simulink model "Model_Linearisierung_final"  (R2023b)
settings: Solver=FixedStepAuto  StartTime=0.0  StopTime=Inf  FixedStep=1e-4  RelTol=1e-3
PostLoadFcn:
  | if any(exist('dsrtsu_mdlpostloadfcn', 'file') ~= 0), dsrtsu_mdlpostloadfcn('Execute', bdroot); end
InitFcn:
  | , if any(exist('rtifpga_mdlclblib', 'file') ~= 0), rtifpga_mdlclblib('Init', bdroot); end,
  | , if any(exist('dsmpb_private', 'file') ~= 0), dsmpb_private('dsmpb_mdlclblib', 'Init', bdroot); end,
  | load('LUT_BRUSA_jax_grad.mat')
  | load('daten_nichtlinear_interpoliert.mat')
  | load('Maschinendaten.mat')
values from neighbouring files (symbols this model uses):
  delta_id = id_fine(2)-id_fine(1)    [Messdaten_Interpoliert.m]    (also in daten_nichtlinear_interpoliert.mat = 2.52525252525)
  delta_iq = iq_fine(2)-iq_fine(1)    [Messdaten_Interpoliert.m]    (also in daten_nichtlinear_interpoliert.mat = 5.05050505051)
  I_max = 170    [Maschinendaten.mat]    (also in Maschinendaten_Vorgabe.m; test_ModelParameters.m = evalin('base', 'I_max'); test_StrategySelection.m = tc.readConstant(tc.BLK_Imax))
  ID = [-250 -250 -250 -250 -250 -250 -250 -250 -250 -250 -250 -250 ... (10000 elements, 100x100)]    [daten_nichtlinear_interpoliert.mat]
  id_fine = linspace(min(id_vec), max(id_vec), 100)    [Messdaten_Interpoliert.m]    (also in daten_nichtlinear_interpoliert.mat = [-250 -247.474747475 -244.949494949 -242.424242424 -239.8989)
  IQ = [-250 -244.949494949 -239.898989899 -234.848484848 -229.797979798 -224.747474747 -219.696969697 -214.646464646 -209.595959596 -204.545454545 -199.494949495 -194.444444444 ... (10000 elements, 100x100)]    [daten_nichtlinear_interpoliert.mat]
  iq_fine = linspace(min(iq_vec), max(iq_vec), 100)    [Messdaten_Interpoliert.m]    (also in daten_nichtlinear_interpoliert.mat = [-250 -244.949494949 -239.898989899 -234.848484848 -229.7979)
  Ldd = Ldd_fine    [Messdaten_Interpoliert.m]    (also in daten_nichtlinear_interpoliert.mat = [0.000225276031415 0.000225750625371 0.000226241749969 0.000)
  Ldq = Ldq_fine    [Messdaten_Interpoliert.m]    (also in daten_nichtlinear_interpoliert.mat = [1.31113456519e-05 1.34236782585e-05 1.31001168558e-05 1.236)
  Lqd = Lqd_fine    [Messdaten_Interpoliert.m]    (also in daten_nichtlinear_interpoliert.mat = [7.22855329514e-05 7.00325573553e-05 6.7613098921e-05 6.5016)
  Lqq = Lqq_fine    [Messdaten_Interpoliert.m]    (also in daten_nichtlinear_interpoliert.mat = [0.000286039721686 0.000286453471045 0.000286025480511 0.000)
  n_max = 11000    [Maschinendaten.mat]    (also in Maschinendaten_Vorgabe.m; test_ModelParameters.m = evalin('base', 'n_max'); test_StrategySelection.m = tc.readConstant(tc.BLK_nmax))
  p = 3    [Maschinendaten.mat]    (also in Maschinendaten_Vorgabe.m; Messdaten_Interpoliert.m; test_ModelParameters.m = evalin('base', 'p'))
  Psid = Psid_fine    [Messdaten_Interpoliert.m]    (also in daten_nichtlinear_interpoliert.mat = [0.00602681114795 0.00609490588107 0.00615917040906 0.006219)
  Psiq = Psiq_fine    [Messdaten_Interpoliert.m]    (also in daten_nichtlinear_interpoliert.mat = [-0.166252688687 -0.164805403122 -0.163363500753 -0.16192610)
  Rs = 0.018    [Maschinendaten.mat]    (also in Maschinendaten_Vorgabe.m; test_ModelParameters.m = evalin('base', 'Rs'))
  U_dc = 560    [Maschinendaten.mat]    (also in Maschinendaten_Vorgabe.m; test_ModelParameters.m = evalin('base', 'U_dc'))
  U_max = 323.316150746    [Maschinendaten.mat]    (also in Maschinendaten_Vorgabe.m = U_dc / sqrt(3); test_ModelParameters.m = evalin('base', 'U_max'))
(part 2 of 3)

== matlab function Model_Linearisierung_final/Subsystem Arbeitspunktsteuerung/Arbeitspunktsteuerung/Glac - Schnittpunktsuche ==
  data: q_current input double size=[1 6]; q_voltage input double size=[1 6]; q_torque input size=[1 6]; q_MTPC input double size=[1 6]; q_MTPV input double size=[1 6]; Imax input size=1; i_ac output size=[4 2]; i_vv output size=[4 2]; i_av output size=[4 2]; i_cv output size=[4 2]; i_at output size=[4 2]; i_tv output size=[4 2]
function [i_ac, i_vv, i_av, i_cv, i_at, i_tv] = ...
    Glac_Block(q_current, q_voltage, q_torque, q_MTPC, q_MTPV, Imax)

%#codegen
coder.extrinsic('disp');
% ================================================================
% GLAC – Schnittpunktbestimmung zweier Quadriken
%
% Eingänge:
%   q_current : Stromkreis
%   q_voltage : Spannungsgrenze
%   q_torque  : Drehmomentkennlinie
%   q_MTPC    : MTPC
%   q_MTPV    : MTPV
%   Imax      : maximaler Strom
%
% Jede Quadrik:
%   q = [a b c d e f]
%
% F(id,iq) =
%   a*id^2 + b*id*iq + c*iq^2 + d*id + e*iq + f
%
% Ausgänge:
%   jeweils 4x2
%
%   [id1 iq1
%    id2 iq2
%    id3 iq3
%    id4 iq4]
%
% Nicht vorhandene Schnittpunkte = NaN
% ================================================================


%% 1. Schnittpunkte bestimmen

% MTPC ∩ Stromkreis
i_ac = intersectGlac(q_MTPC, q_current, Imax);

% MTPV ∩ Spannung
i_vv = intersectGlac(q_MTPV, q_voltage, Imax);

% MTPC ∩ Spannung
i_av = intersectGlac(q_MTPC, q_voltage, Imax);

% Stromkreis ∩ Spannung
i_cv = intersectGlac(q_current, q_voltage, Imax);

% MTPC ∩ Drehmoment
i_at = intersectGlac(q_MTPC, q_torque, Imax);

% Drehmoment ∩ Spannung
i_tv = intersectGlac(q_torque, q_voltage, Imax);

disp('--- Schnittpunkte: i_ac, i_vv, i_av, i_cv, i_at, i_tv ---');
disp('i_ac:');
disp(i_ac);
disp('i_vv:');
disp(i_vv);
disp('i_av:');
disp(i_av);
disp('i_cv:');
disp(i_cv);
disp('i_at:');
disp(i_at);
disp('i_tv:');
disp(i_tv);
end

%%%%%%%%%%%%%%%%%%%%%%%%%%%%%%%%%%%%%%%%%%%%%%%%%%%%%%%%%%%%%%%%%%%%%%%%%%%
%% GLAC-SCHNITTPUNKTSUCHE ==> Überprüft !
% Analytische Schnittpunktbestimmung zweier Quadriken nach Glac
%
% Eingabe:
%   qA, qB : Quadrikkoeffizienten [a b c d e f]
%            F(id, iq) = a*id^2 + b*id*iq + c*iq^2 + d*id + e*iq + f = 0
%   Imax   : Maximaler Strom zur Normierung [A]
%
% Ausgabe:
%   pts    : 4x2 Matrix mit [id, iq]-Schnittpunkten, sortiert nach
%            dem Glac-Gütefaktor s = idN^2 + 0.1*iqN^2.
%            Nicht existierende Schnittpunkte sind mit NaN befüllt.

function pts = intersectGlac(qA, qB, Imax)

    % ---Ausgabe immer 4x2 ---------------------------------------------------
    pts = NaN(4, 2);
    ZERO_TOL = 1e-12; % Glac Toleranz für Null-Konstante 9.0e-4 -> ggf 1e-10

    %% 1. Normierung der Quadriken auf Imax
    A = zeros(1, 6);
    B = zeros(1, 6);
    A(1) = qA(1); 
    A(2) = qA(2); 
    A(3) = qA(3); 
    A(4) = qA(4)/Imax; 
    A(5) = qA(5)/Imax; 
    A(6) = qA(6)/(Imax*Imax);
    B(1) = qB(1); 
    B(2) = qB(2); 
    B(3) = qB(3); 
    B(4) = qB(4)/Imax; 
    B(5) = qB(5)/Imax; 
    B(6) = qB(6)/(Imax*Imax);

    %% 2. Transformation in Glac-Matrixdarstellung
    % F = x11*x1^2 + 2*x12*x1*x2 + x22*x2^2 + 2*x1*x1 + 2*x2*x2 + x0
    M_A_x11 = A(1); 
    M_A_x12 = A(2)/2; 
    M_A_x22 = A(3); 
    M_A_x1  = A(4)/2; 
    M_A_x2  = A(5)/2; 
    M_A_x0  = A(6);

    M_B_x11 = B(1); 
    M_B_x12 = B(2)/2; 
    M_B_x22 = B(3); 
    M_B_x1  = B(4)/2; 
    M_B_x2  = B(5)/2; 
    M_B_x0  = B(6);


    %% 3. Fallunterscheidung zur Bildung der Matrizen D und M
    translate = false;

    if (abs(M_A_x0) > ZERO_TOL) && (abs(M_B_x0) > ZERO_TOL)
        % Fall 1: Beide Konstantenterme != 0
        a0inv = 1 / M_A_x0;
        b0inv = 1 / M_B_x0;

        D_x11 = M_A_x11*a0inv - M_B_x11*b0inv;
        D_x12 = M_A_x12*a0inv - M_B_x12*b0inv;
        D_x22 = M_A_x22*a0inv - M_B_x22*b0inv;
        D_x1  = M_A_x1*a0inv  - M_B_x1*b0inv;
        D_x2  = M_A_x2*a0inv  - M_B_x2*b0inv;

        if abs(a0inv) > abs(b0inv)
            M_x11 = M_B_x11; M_x12 = M_B_x12; M_x22 = M_B_x22;
            M_x1  = M_B_x1;  M_x2  = M_B_x2;  M_x0  = M_B_x0;
        else
            M_x11 = M_A_x11; M_x12 = M_A_x12; M_x22 = M_A_x22;
            M_x1  = M_A_x1;  M_x2  = M_A_x2;  M_x0  = M_A_x0;
        end

    elseif (abs(M_A_x0) <= ZERO_TOL) && (abs(M_B_x0) > ZERO_TOL)
        % Fall 2: A.x0 == 0, B.x0 != 0
        D_x11 = M_A_x11; D_x12 = M_A_x12; D_x22 = M_A_x22;
        D_x1  = M_A_x1;  D_x2  = M_A_x2;
        M_x11 = M_B_x11; M_x12 = M_B_x12; M_x22 = M_B_x22;
        M_x1  = M_B_x1;  M_x2  = M_B_x2;  M_x0  = M_B_x0;

    elseif (abs(M_A_x0) > ZERO_TOL) && (abs(M_B_x0) <= ZERO_TOL)
        % Fall 3: A.x0 != 0, B.x0 == 0
        D_x11 = M_B_x11; D_x12 = M_B_x12; D_x22 = M_B_x22;
        D_x1  = M_B_x1;  D_x2  = M_B_x2;
        M_x11 = M_A_x11; M_x12 = M_A_x12; M_x22 = M_A_x22;
        M_x1  = M_A_x1;  M_x2  = M_A_x2;  M_x0  = M_A_x0;

    else
        % Fall 4: Beide x0 == 0 -> Translation
        xs1 = 0.5;
        xs2 = 0.3;

        alfa_s = 2*M_A_x1*xs1 + 2*M_A_x2*xs2 + ...
                 xs1*(M_A_x11*xs1 + M_A_x12*xs2) + ...
                 xs2*(M_A_x12*xs1 + M_A_x22*xs2);

        beta_s = 2*M_B_x1*xs1 + 2*M_B_x2*xs2 + ...
                 xs1*(M_B_x11*xs1 + M_B_x12*xs2) + ...
                 xs2*(M_B_x12*xs1 + M_B_x22*xs2);

        if abs(alfa_s) < 1e-12 || abs(beta_s) < 1e-12
            return;
        end

        alfa_s_inv = 1 / alfa_s;
        beta_s_inv = 1 / beta_s;

        D_x11 = M_A_x11*alfa_s_inv - M_B_x11*beta_s_inv;
        D_x12 = M_A_x12*alfa_s_inv - M_B_x12*beta_s_inv;
        D_x22 = M_A_x22*alfa_s_inv - M_B_x22*beta_s_inv;

        D_x1 = (M_A_x1 + M_A_x11*xs1 + M_A_x12*xs2)*alfa_s_inv - ...
               (M_B_x1 + M_B_x11*xs1 + M_B_x12*xs2)*beta_s_inv;

        D_x2 = (M_A_x2 + M_A_x12*xs1 + M_A_x22*xs2)*alfa_s_inv - ...
               (M_B_x2 + M_B_x12*xs1 + M_B_x22*xs2)*beta_s_inv;

        M_x11 = M_B_x11; M_x12 = M_B_x12; M_x22 = M_B_x22;
        M_x1  = M_B_x1 + M_B_x11*xs1 + M_B_x12*xs2;
        M_x2  = M_B_x2 + M_B_x12*xs1 + M_B_x22*xs2;
        M_x0  = beta_s;

        translate = true;
    end

    if abs(M_x0) < 1e-14
        return;
    end


 %% 4. Aufstellen des Quartik-Polynoms in xi
    invM0 = 1 / M_x0;
    xi4 = 1.0;
    xi3 = invM0 * (4*D_x2*M_x1 - 4*D_x1*M_x2);
    xi2 = invM0 * (4*D_x2^2*M_x11 + 4*D_x1^2*M_x22 - 2*D_x12^2*M_x0 ...
                 - 8*D_x1*D_x2*M_x12 + 4*D_x1*D_x12*M_x2 - 4*D_x2*D_x11*M_x2 ...
                 + 4*D_x2*D_x12*M_x1 - 4*D_x1*D_x22*M_x1 + 2*D_x11*D_x22*M_x0);
    xi1 = invM0 * (4*D_x1*D_x12^2*M_x2 - 4*D_x2*D_x12^2*M_x1 ...
                 - 8*D_x2^2*D_x11*M_x12 + 8*D_x2^2*D_x12*M_x11 ...
                 - 8*D_x1^2*D_x12*M_x22 + 8*D_x1^2*D_x22*M_x12 ...
                 + 8*D_x1*D_x2*D_x11*M_x22 - 8*D_x1*D_x2*D_x22*M_x11 ...
                 - 4*D_x1*D_x11*D_x22*M_x2 + 4*D_x2*D_x11*D_x22*M_x1);
    xi0 = invM0 * (D_x12^4*M_x0 + 4*D_x2^2*D_x12^2*M_x11 + 4*D_x1^2*D_x22^2*M_x11 ...
                 + 4*D_x1^2*D_x12^2*M_x22 + 4*D_x2^2*D_x11^2*M_x22 + D_x11^2*D_x22^2*M_x0 ...
                 - 4*D_x1*D_x12^3*M_x2 - 4*D_x2*D_x12^3*M_x1 + 8*D_x1*D_x2*D_x12^2*M_x12 ...
                 + 4*D_x2*D_x11*D_x12^2*M_x2 - 4*D_x1*D_x11*D_x22^2*M_x1 ...
                 + 4*D_x1*D_x12^2*D_x22*M_x1 - 4*D_x2*D_x11^2*D_x22*M_x2 ...
                 - 8*D_x2^2*D_x11*D_x12*M_x12 - 8*D_x1^2*D_x12*D_x22*M_x12 ...
                 - 2*D_x11*D_x12^2*D_x22*M_x0 - 8*D_x1*D_x2*D_x11*D_x12*M_x22 ...
                 + 8*D_x1*D_x2*D_x11*D_x22*M_x12 - 8*D_x1*D_x2*D_x12*D_x22*M_x11 ...
                 + 4*D_x1*D_x11*D_x12*D_x22*M_x2 + 4*D_x2*D_x11*D_x12*D_x22*M_x1);

 

    %% 5. Quartik lösen
    xiRoots = roots([xi4, xi3, xi2, xi1, xi0]);
    
    disp('xiRoots:');
    disp(xiRoots);

    %% 6. Rekonstruktion der Schnittpunkte (id, iq)
    validCount = 0;
    tempPts = NaN(4, 2);
    tempSort = NaN(4, 1);

    for k = 1:numel(xiRoots)
        xi = xiRoots(k);

        % Nur reelle Nullstellen verarbeiten
        if abs(imag(xi)) < 1e-6
            xi_r = real(xi);
            denXi = xi_r^2 + D_x11*D_x22 - D_x12^2;

            if abs(denXi) > 1e-12
                adjXi = 1 / denXi;

                if translate
                    xs1 = 0.5; xs2 = 0.3;
                    idN = -2*adjXi*(D_x22*D_x1 + (-D_x12 - xi_r)*D_x2) + xs1;
                    iqN = -2*adjXi*((xi_r - D_x12)*D_x1 + D_x11*D_x2) + xs2;
                else
                    idN = -2*adjXi*(D_x22*D_x1 + (-D_x12 - xi_r)*D_x2);
                    iqN = -2*adjXi*((xi_r - D_x12)*D_x1 + D_x11*D_x2);
                end

                if abs(imag(idN)) < 1e-6 && abs(imag(iqN)) < 1e-6
                    idN = real(idN);
                    iqN = real(iqN);

                    id = idN * Imax;
                    iq = iqN * Imax;

                    % Residuen-Prüfung gegen ursprüngliche Quadriken
                    resA = qA(1)*id^2 + qA(2)*id*iq + qA(3)*iq^2 + qA(4)*id + qA(5)*iq + qA(6);
                    resB = qB(1)*id^2 + qB(2)*id*iq + qB(3)*iq^2 + qB(4)*id + qB(5)*iq + qB(6);
                    
                    scaleA = abs(qA(1)*id^2) + abs(qA(2)*id*iq) + abs(qA(3)*iq^2) + abs(qA(4)*id) + abs(qA(5)*iq) + abs(qA(6)) + 1;
                    scaleB = abs(qB(1)*id^2) + abs(qB(2)*id*iq) + abs(qB(3)*iq^2) + abs(qB(4)*id) + abs(qB(5)*iq) + abs(qB(6)) + 1;

                    disp('xi =');
                    disp(xi_r);
                    disp('idN =');
                    disp(idN);
                    disp(' iqN =');
                    disp(iqN);
                    disp('resA = ');
                    disp(abs(resA)/scaleA);
                    disp('resB = ');
                    disp(abs(resB)/scaleB);

                    if (abs(resA)/scaleA < 1e-2) && (abs(resB)/scaleB < 1e-2)
                        validCount = validCount + 1;
                        tempPts(validCount, :) = [id, iq];
                        tempSort(validCount) = idN^2 + 0.1*iqN^2; % Glac Sortierkriterium
                    end
                end
            end
        end
    end

    %% 7. Aufsteigend nach Glac-Gütekriterium sortieren
    if validCount > 0
        [~, idx] = sort(tempSort(1:validCount), 'ascend');
        for i = 1:validCount
            pts(i, :) = tempPts(idx(i), :);
        end
    end
end

== matlab function Model_Linearisierung_final/Subsystem Arbeitspunktsteuerung/Vorläufiger Arbeitspunkt aus alter Steuerug/Kennfelder/ Vorberechnung gemeinsamer Größen ==
  data: ID input; IQ input; Ld input; Lq input; Lm input; PSID input; PSIQ input; Rs input; omega input; p input; I_max input; U_max input; Ldq output; Ldq_p output; Ld_q output; Lq_d output; Ld2 output; Lq2 output; Lm2 output; psid1 output; psiq1 output; omega2 output; Rs2 output; stromgrenze output; spannungsgrenze output; I_max2 output; U_max2 output; psi2 output; T_ref output; T_feld output; T_soll input
%% 4) Vorberechnung gemeinsamer Größen
% Dieser Block dient der Laufzeitoptimierung.
% Alle häufig benötigten Terme werden einmal zentral berechnet und später
% wiederverwendet. So werden Mehrfachrechnungen vermieden.

function [Ldq, Ldq_p, Ld_q, Lq_d, Ld2, Lq2, Lm2, psid1, psiq1, omega2, Rs2, stromgrenze, spannungsgrenze, I_max2, U_max2, psi2, T_ref, T_feld] = fcn(ID, IQ, Ld, Lq, Lm, PSID, PSIQ, Rs, omega, p, I_max, U_max, T_soll)

% Strom und Spannungsgrenzen
ID2   = ID.^2;
IQ2   = IQ.^2;
IDIQ  = ID.*IQ;

% Maschinenparameter
Ldq = Ld - Lq;      % Differenz Ld - Lq
Ldq_p = Ld + Lq;    % Summe Ld + Lq
Ld_q = Ld.*Lq;      % Matrixmultiplikation Ld.* Lq
Lq_d = Lq.*Ld;      % Matrixmultiplikation Lq.* Ld
Ld2 = Ld.^2;        % Quadrat Ld
Lq2 = Lq.^2;        % Quadrat Lq
Lm2 = Lm.^2;        % Quadrat Lm
psid1 = 1.5*p*PSID; % Vorfaktor PSID
psiq1 = 1.5*p*PSIQ; % Vorfaktor PSIQ
omega2 = omega^2;   % Quadrat Omega
Rs2 = Rs^2;         % Quadrat Rs

% Spannungsanteile in d- und q-Richtung
ud = Rs .* ID - omega .* PSIQ;
uq = Rs .* IQ + omega .* PSID;

% Quadrat von Strom- und Spannungsbetrag
I2 = ID2 + IQ2;
U2 = ud.^2 + uq.^2;

I_max2 = I_max^2;
U_max2 = U_max^2;

% Grenzfunktionen:
stromkreis = I2 - I_max2; % Stromkreis (Betragsgrenze)
spannung   = U2 - U_max2; % Spannungsellipse
stromgrenze = stromkreis;
spannungsgrenze = spannung;

% Flussbetrag
psi2 = PSID.^2 + PSIQ.^2;

% Drehmoment
T_feld = 3/2*p*(PSID.*IQ - PSIQ.*ID);

% Referenz-Drehmomenthyperbel
T_ref = T_feld - T_soll;

== matlab function Model_Linearisierung_final/Subsystem Arbeitspunktsteuerung/Vorläufiger Arbeitspunkt aus alter Steuerug/Kennfelder/MTPC-Kennlinie ==
  data: psid1 input; psiq1 input; Lm input; f_MTPC output; Ldq input; p input; ID input; IQ input
%% MTPC Kennlinie 
% konstant, da nur abhängig von Induktivitäten und Flüssen  
function f_MTPC = fcn(psid1, psiq1, Lm, Ldq, p, ID, IQ)

%Psi_pm = 0.068; 
M11 = (Ldq)./2;
M12 = Lm;
M22 = -(Ldq)./2;
mc1 = psid1./4;
mc2 = psiq1./4;

f_MTPC = 1.5*p*(M11.*ID.^2 + 2*M12.*ID.*IQ + M22.*IQ.^2)...
         + 2*(mc1.*ID + mc2.*IQ);

== matlab function Model_Linearisierung_final/Subsystem Arbeitspunktsteuerung/Vorläufiger Arbeitspunkt aus alter Steuerug/Kennfelder/MTPF-Kennlinie ==
  data: Lm input; f_MTPF output; Ld input; Lq input; Ldq input; Ldq_p input; Ld2 input; Lq2 input; Ld_q input; Lq_d input; Lm2 input; PSID input; PSIQ input; p input; ID input; IQ input
%% MTPF Kennlinie 
% konstant, da nur abhängig von Induktivitäten und Flüssen
function f_MTPF = fcn(Lm, Ld, Lq, Ldq, Ldq_p, Ld2, Lq2, Ld_q, Lq_d, Lm2, PSID, PSIQ, p, ID, IQ)

Mf11 = (Ldq)./2 .*(Ld2 + Lm2) + Lm2 .*(Ldq_p);
Mf12 = Lm./2.*(Ld2 + Lq2 + 2*Lm2);
Mf22 = -(Ldq)./2 .*(Lq2 + Lm2) + Lm2 .*(Ldq_p);

mf1 = 1.5*p*((2*Ld2 - Lq_d + 3*Lm2).*PSID./4 ...
      + Lm.* (Ldq_p).*PSIQ./2);
mf2 = 1.5*p*(Lm.* (Ldq_p).*PSID./2 ...
      + (2*Lq2 - Ld_q + 3*Lm2).*PSIQ./4);

my_f = 0.75*p*(Ld.*(PSID).^2 + 2*Lm.*PSID.*PSIQ + Lq.*(PSIQ).^2);

f_MTPF = 1.5*p*(Mf11.*ID.^2 + 2*Mf12.*ID.*IQ + Mf22.*IQ.^2)...
         + 2*(mf1.*ID + mf2.*IQ) + my_f;

== matlab function Model_Linearisierung_final/Subsystem Arbeitspunktsteuerung/Vorläufiger Arbeitspunkt aus alter Steuerug/Kennfelder/MTPV-Kennlinie ==
  data: Lm input; f_MTPV output; Ld input; Lq input; Lm2 input; Ld2 input; Lq2 input; Ldq input; Ldq_p input; Lq_d input; PSID input; PSIQ input; p input; omega2 input; ID input; IQ input; Rs2 input
%% MTPV Kennlinie 
% Ändert sich mit Drehzahl omega
function f_MTPV = fcn(Lm, Ld, Lq, Lm2, Ld2, Lq2, Ldq, Ldq_p, Lq_d, PSID, PSIQ, p, omega2, ID, IQ, Rs2)

Mv11 = omega2*Lm2.*(Ldq_p)...
       + (Ldq)./2 .*(Rs2 + omega2*(Ld2 + Lm2));
Mv12 = Lm./2.*(2*Rs2+omega2*(Ld2 + Lq2 + 2*Lm2));
Mv22 = omega2*Lm2.*(Ldq_p)...
       - (Ldq)./2 .*(Rs2 + omega2*(Lq2 + Lm2));
mv1 = 1.5*p*((Rs2 + omega2* (2*Ld2 - Lq_d + 3*Lm2)).*PSID./4 ... 
      + omega2*Lm.* (Ldq_p).*PSIQ./2);
mv2 = 1.5*p*(omega2*Lm.* (Ldq_p).*PSID./2 ...
      + (Rs2 + omega2*(2*Ld2 - Lq_d + 3*Lm2)).*PSIQ./4);
my_v = 0.75*p*omega2*(Ld.*(PSID).^2 + 2*Lm.*PSID.*PSIQ + Lq.*(PSIQ).^2);

f_MTPV = 1.5*p*(Mv11.*ID.^2 + 2*Mv12.*ID.*IQ + Mv22.*IQ.^2)...
         + 2*(mv1.*ID + mv2.*IQ) + my_v;

== matlab function Model_Linearisierung_final/Subsystem Arbeitspunktsteuerung/Vorläufiger Arbeitspunkt aus alter Steuerug/Strategieauswahl und Arbeitspunkt id*, iq* ==
  data: n_mech input; n_max input; T_soll input; T_feld input; T_ref input; signT input; id_fine input; iq_fine input; I_max2 input; U_max2 input; stromkreis input; spannung input; psi2 input; f_MTPC input; f_MTPV input; f_MTPF input; id_ref output; iq_ref output; out_iat output; out_itv output; out_iac output; out_icv output; feasCode output; boundaryCode output
%% Strategieauswahl gemäß Flowchart und Bestimmung Arbeitspunkt id*, iq*
% Interpolation, Charak. Punkte, Flowchart-Logik, Nachverfeinerung

function [id_ref, iq_ref, out_iat, out_itv, out_iac, out_icv, feasCode, boundaryCode] = fcn( ...
     n_mech, n_max, T_soll, T_feld, T_ref, signT,...
     id_fine, iq_fine, I_max2, U_max2, ...
     stromkreis,spannung, psi2, f_MTPC, f_MTPV, f_MTPF)

% Strategiecodes, da keine Textausgabe möglich:
% Fälle:
%   out_iat = 1  -> MTPC ∩ T_soll, Sollmoment erreichbar
%   out_itv = 1  -> U_max ∩ T_soll, Sollmoment erreichbar
%   out_iac = 1  -> MTPC ∩ I_max, Sollmoment nicht erreichbar
%   out_icv = 1  -> I_max ∩ U_max, Sollmoment nicht erreichbar
%
% feasCode:
% 0 = none
% 1 = i_vv
% 2 = i_ac
% 3 = i_cv
%
% boundaryCode:
% 0 = none
% 1 = voltage boundary
% 2 = current boundary

%% Konstanten fuer Root-/Mode-Codes
ROOT_AC = 1;
ROOT_VV = 2;
ROOT_AV = 3;
ROOT_CV = 4;
ROOT_AT = 5;
ROOT_TV = 6;

MODE_INTERIOR = 1;
MODE_BOUNDARY = 2;
MODE_VOLTAGE  = 3;

BND_NONE    = 0;
BND_VOLTAGE = 1;
BND_CURRENT = 2;

%% Initialisierung
id_ref = 0.0;
iq_ref = 0.0;
feasCode = int32(0);
boundaryCode = int32(0);

i_ref  = [NaN NaN];
i_feas = [NaN NaN];

out_iat = 0.0;
out_itv = 0.0;
out_iac = 0.0;
out_icv = 0.0;

%% Schutz
if n_mech > n_max
    id_ref = 0.0;
    iq_ref = 0.0;
    feasCode = int32(0);
    boundaryCode = int32(0);
    return;
end

%% 4) Kontext
ctx.xvec   = id_fine;
ctx.yvec   = iq_fine;
ctx.Ti     = T_feld;
ctx.Teql   = T_ref;
ctx.Ieql   = stromkreis;
ctx.Ueql   = spannung;
ctx.Psi2i  = psi2;
ctx.MTPCi  = f_MTPC;
ctx.MTPVi  = f_MTPV;
ctx.MTPFi  = f_MTPF;
ctx.Tref   = T_soll;
ctx.signT  = signT;
ctx.tolEq  = 1e-6 * max([1, I_max2, U_max2, abs(T_soll)]);
ctx.tolT   = max(0.25, 1e-3*max(1, abs(T_soll)));

%% 5) Charakteristische Punkte im Flowchart
pts_iac = findCurveIntersections(id_fine, iq_fine, f_MTPC,    0.0, stromkreis, 0.0, ctx);
pts_ivv = findCurveIntersections(id_fine, iq_fine, f_MTPV,    0.0, spannung,   0.0, ctx);
pts_iav = findCurveIntersections(id_fine, iq_fine, f_MTPC,    0.0, spannung,   0.0, ctx);
pts_icv = findCurveIntersections(id_fine, iq_fine, stromkreis,0.0, spannung,   0.0, ctx);
pts_iat = findCurveIntersections(id_fine, iq_fine, f_MTPC,    0.0, T_ref,  0.0, ctx);
pts_itv = findCurveIntersections(id_fine, iq_fine, T_ref, 0.0, spannung,   0.0, ctx);

i_ac = chooseCorrectRoot(pts_iac, ROOT_AC, ctx);
i_vv = chooseCorrectRoot(pts_ivv, ROOT_VV, ctx);
i_av = chooseCorrectRoot(pts_iav, ROOT_AV, ctx);
i_cv = chooseCorrectRoot(pts_icv, ROOT_CV, ctx);
i_at = chooseCorrectRoot(pts_iat, ROOT_AT, ctx);
i_tv = chooseCorrectRoot(pts_itv, ROOT_TV, ctx);

%% 6) Flowchart-Logik
% ------------------------------------------------------------
% Fall 1: MTPC ∩ T_soll -> i_at
% Nur wenn Sollmoment auf dem MTPC-Zweig noch erreichbar ist
% ------------------------------------------------------------

if isFinitePoint(i_at)
    I_at = evalGI(ctx.Ieql, i_at, ctx);
    U_at = evalGI(ctx.Ueql, i_at, ctx);

    if (I_at <= 1e-5) && (U_at <= 1e-5)
        i_ref = finalFeasiblePolish(i_at, MODE_INTERIOR, ctx);
        out_iat = 1;    % Sollmoment T* auf MTPC
    end
end

% --- falls MTPC ∩ T_soll nicht direkt zulässig ---
if ~isFinitePoint(i_ref)
    % i_feas bestimmen:
    % Vergleich psi_cv und psi_ac:
    %    - psi_cv > psi_ac  -> i_feas = i_ac
    %    - sonst            -> i_feas = i_cv

    if isFinitePoint(i_vv) && evalGI(ctx.Ieql, i_vv, ctx) <= 1e-5
        i_feas = i_vv;
        feasCode = int32(1); % 1 = i_vv
    else
        psi_ac = inf;
        psi_cv = inf;

        if isFinitePoint(i_ac)
            psi_ac = sqrt(max(evalGI(ctx.Psi2i, i_ac, ctx), 0.0));
        end
        if isFinitePoint(i_cv)
            psi_cv = sqrt(max(evalGI(ctx.Psi2i, i_cv, ctx), 0.0));
        end

        if psi_cv > psi_ac
            i_feas = i_ac;
            feasCode = int32(2); % 2 = i_ac
        else
            i_feas = i_cv;
            feasCode = int32(3); % 3 = i_cv
        end
    end

    m_av  = NaN;
    m_max = NaN;

    if isFinitePoint(i_av)
        m_av = evalGI(ctx.Ti, i_av, ctx);
    end
    if isFinitePoint(i_feas)
        m_max = evalGI(ctx.Ti, i_feas, ctx);
    end

    % ------------------------------------------------------------
    % Fall 2: U_max ∩ T_soll  -> i_tv
    % Sollmoment ist auf der Spannungsgrenze noch erreichbar
    % ------------------------------------------------------------
    if isFinitePoint(i_tv) && isfinite(m_max) && abs(T_soll) <= abs(m_max) + ctx.tolT
        i_ref = finalFeasiblePolish(i_tv, MODE_VOLTAGE, ctx);
        out_itv = 1;    % Sollmoment T* auf Umax 
    end

    % ------------------------------------------------------------
    % Fall 3: MTPC ∩ I_max -> i_ac
    % Sollmoment nicht mehr erreichbar, Umschalten auf Stromgrenze
    % sonst: 
    % Fall 4: I_max ∩ U_max -> i_cv
    % Sollmoment nicht mehr erreichbar, Spannungs- und Stromgrenze aktiv
    % ------------------------------------------------------------
    if ~isFinitePoint(i_ref) && isFinitePoint(i_feas)
        i_ref = i_feas;

        if feasCode == int32(2)
            out_iac = 1;        % KEIN Sollmoment T*, Arbeitspunkt auf MTPC bei Imax
        elseif feasCode == int32(3)
            out_icv = 1;        % KEIN Sollmoment T*,  ARbeitspunkt am Schnittpunkt Imax und Umax
        end
    end
end

%% 7) Schluss-Nachverfeinerung
if isFinitePoint(i_ref)
   if out_itv == 1
       i_ref = refineOnBoundary(i_ref, BND_VOLTAGE, ctx);
  elseif out_iat == 1
       i_ref = finalFeasiblePolish(i_ref, MODE_INTERIOR, ctx);

   elseif out_iac == 1 || out_icv == 1
      % Saettigungs- bzw. Grenzpunkt nicht unnoetig wegziehen
 end
end

%% 8) Ausgaenge
if isFinitePoint(i_ref)
    id_ref = i_ref(1);
    iq_ref = i_ref(2);
else
    id_ref = 0.0;
    iq_ref = 0.0;
end

end

%% == lokale Hilfsfunktionen ===========================================

function z = evalGI(G, p, ctx)
    z = interp2_bilinear_clamped(ctx.xvec, ctx.yvec, G, p(1), p(2));
end

% ========================================================================
function tf = isFinitePoint(p)
    tf = isnumeric(p) && numel(p)==2 && all(isfinite(p));
end

% ========================================================================
function pts = findCurveIntersections(xvec, yvec, F1, lev1, F2, lev2, ctx)

    MAX_PTS = 24;
    pts = nan(MAX_PTS, 2);
    nPts = 0;

    A = F1 - lev1;
    B = F2 - lev2;

    nx = numel(xvec);
    ny = numel(yvec);

    dxMin = min(abs(diff(xvec)));
    dyMin = min(abs(diff(yvec)));
    tolMerge = 0.25 * min(dxMin, dyMin);

    scaleA = max(1.0, max(abs(A(:))));
    scaleB = max(1.0, max(abs(B(:))));
    tolRes = 1e-4;

    for r = 1:ny-1
        for c = 1:nx-1

            Ac = [A(r,c), A(r,c+1), A(r+1,c), A(r+1,c+1)];
            Bc = [B(r,c), B(r,c+1), B(r+1,c), B(r+1,c+1)];

            crossA = (min(Ac) <= 0) && (max(Ac) >= 0);
            crossB = (min(Bc) <= 0) && (max(Bc) >= 0);

            if ~(crossA && crossB)
                continue;
            end

            x0 = 0.5 * (xvec(c) + xvec(c+1));
            y0 = 0.5 * (yvec(r) + yvec(r+1));
            p0 = [x0, y0];

            p1 = localRefine2D(p0, A, B, xvec, yvec, 4, 11);
            p2 = localRefineGN(p1, A, B, xvec, yvec);

            a2 = interp2_bilinear_clamped(xvec, yvec, A, p2(1), p2(2)) / scaleA;
            b2 = interp2_bilinear_clamped(xvec, yvec, B, p2(1), p2(2)) / scaleB;
            res = sqrt(a2*a2 + b2*b2);

            if res < tolRes
                if ~pointExists(pts, p2, tolMerge)
                    nPts = nPts + 1;
                    if nPts <= MAX_PTS
                        pts(nPts,:) = p2;
                    end
                end
            end
        end
    end

    for k = 1:MAX_PTS
        if all(isfinite(pts(k,:)))
            v1 = evalGI(A, pts(k,:), ctx);
            v2 = evalGI(B, pts(k,:), ctx);
            if ~(isfinite(v1) && isfinite(v2))
                pts(k,:) = [NaN NaN];
            end
        end
    end
end

% ========================================================================
function tf = pointExists(pts, p, tol)
    tf = false;
    for k = 1:size(pts,1)
        if all(isfinite(pts(k,:)))
            d = hypot(pts(k,1)-p(1), pts(k,2)-p(2));
            if d <= tol
                tf = true;
                return;
            end
        end
    end
end

% ========================================================================
function xBest = localRefine2D(x0, F1i, F2i, xvec, yvec, nIter, nGrid)

    xBest = x0(:).';

    dx0 = min(abs(diff(xvec)));
    dy0 = min(abs(diff(yvec)));

    hx = 2*dx0;
    hy = 2*dy0;

    s1 = max(1.0, max(abs(F1i(:))));
    s2 = max(1.0, max(abs(F2i(:))));

    for it = 1:nIter
        xL = max(min(xvec), xBest(1)-hx);
        xU = min(max(xvec), xBest(1)+hx);
        yL = max(min(yvec), xBest(2)-hy);
        yU = min(max(yvec), xBest(2)+hy);

        bestE = inf;
        bestX = xBest(1);
        bestY = xBest(2);

        for iy = 0:nGrid-1
            if nGrid == 1
                yq = 0.5*(yL+yU);
            else
                yq = yL + (yU-yL) * (iy/(nGrid-1));
            end

            for ix = 0:nGrid-1
                if nGrid == 1
                    xq = 0.5*(xL+xU);
                else
                    xq = xL + (xU-xL) * (ix/(nGrid-1));
                end

                z1 = interp2_bilinear_clamped(xvec, yvec, F1i, xq, yq) / s1;
                z2 = interp2_bilinear_clamped(xvec, yvec, F2i, xq, yq) / s2;
                E  = z1*z1 + z2*z2;

                if E < bestE
                    bestE = E;
                    bestX = xq;
                    bestY = yq;
                end
            end
        end

        xBest = [bestX, bestY];
        hx = hx/3;
        hy = hy/3;
    end
end

% ========================================================================
function xBest = localRefineGN(x0, F1i, F2i, xvec, yvec)

    x = x0(1);
    y = x0(2);

    lbx = min(xvec); ubx = max(xvec);
    lby = min(yvec); uby = max(yvec);

    dx = min(abs(diff(xvec)));
    dy = min(abs(diff(yvec)));

    sx = max(1e-6, 0.25*dx);
    sy = max(1e-6, 0.25*dy);

    s1 = max(1.0, max(abs(F1i(:))));
    s2 = max(1.0, max(abs(F2i(:))));

    lambda = 1e-6;

    for it = 1:12
        f1 = interp2_bilinear_clamped(xvec, yvec, F1i, x, y) / s1;
        f2 = interp2_bilinear_clamped(xvec, yvec, F2i, x, y) / s2;

        f1xp = interp2_bilinear_clamped(xvec, yvec, F1i, clampScalar(x+sx,lbx,ubx), y) / s1;
        f1xm = interp2_bilinear_clamped(xvec, yvec, F1i, clampScalar(x-sx,lbx,ubx), y) / s1;
        f1yp = interp2_bilinear_clamped(xvec, yvec, F1i, x, clampScalar(y+sy,lby,uby)) / s1;
        f1ym = interp2_bilinear_clamped(xvec, yvec, F1i, x, clampScalar(y-sy,lby,uby)) / s1;

        f2xp = interp2_bilinear_clamped(xvec, yvec, F2i, clampScalar(x+sx,lbx,ubx), y) / s2;
        f2xm = interp2_bilinear_clamped(xvec, yvec, F2i, clampScalar(x-sx,lbx,ubx), y) / s2;
        f2yp = interp2_bilinear_clamped(xvec, yvec, F2i, x, clampScalar(y+sy,lby,uby)) / s2;
        f2ym = interp2_bilinear_clamped(xvec, yvec, F2i, x, clampScalar(y-sy,lby,uby)) / s2;

        j11 = (f1xp - f1xm) / (2*sx);
        j12 = (f1yp - f1ym) / (2*sy);
        j21 = (f2xp - f2xm) / (2*sx);
        j22 = (f2yp - f2ym) / (2*sy);

        h11 = j11*j11 + j21*j21 + lambda;
        h12 = j11*j12 + j21*j22;
        h22 = j12*j12 + j22*j22 + lambda;

        g1 = j11*f1 + j21*f2;
        g2 = j12*f1 + j22*f2;

        detH = h11*h22 - h12*h12;
        if abs(detH) < 1e-16
            break;
        end

        dxStep = -( h22*g1 - h12*g2 ) / detH;
        dyStep = -( -h12*g1 + h11*g2 ) / detH;

        dxStep = clampScalar(dxStep, -dx, dx);
        dyStep = clampScalar(dyStep, -dy, dy);

        xNew = clampScalar(x + dxStep, lbx, ubx);
        yNew = clampScalar(y + dyStep, lby, uby);

        oldObj = f1*f1 + f2*f2;
        nf1 = interp2_bilinear_clamped(xvec, yvec, F1i, xNew, yNew) / s1;
        nf2 = interp2_bilinear_clamped(xvec, yvec, F2i, xNew, yNew) / s2;
        newObj = nf1*nf1 + nf2*nf2;

        if newObj < oldObj
            x = xNew;
            y = yNew;
            lambda = max(1e-10, 0.3*lambda);
        else
            lambda = min(1e2, 10*lambda);
        end

        if hypot(dxStep, dyStep) < 1e-10
            break;
        end
    end

    xBest = [x, y];
end

% ========================================================================
function p = chooseCorrectRoot(points, labelCode, ctx)

    p = [NaN NaN];
    scoreBest = inf;

    for k = 1:size(points,1)
        x = points(k,:);
        if ~all(isfinite(x))
            continue;
        end

        Te = evalGI(ctx.Ti,   x, ctx);
        Ie = evalGI(ctx.Ieql, x, ctx);
        Ue = evalGI(ctx.Ueql, x, ctx);
        ps = sqrt(max(evalGI(ctx.Psi2i, x, ctx),0.0));
        iq = x(2);
        Iabs = hypot(x(1), x(2));

        branchPenalty = 0.0;
        if sign(iq) ~= ctx.signT
            branchPenalty = 100.0;
        end

        feasiblePenalty = 0.0;
        if Ie > 1e-6
            feasiblePenalty = feasiblePenalty + 10.0*Ie;
        end
        if Ue > 1e-6
            feasiblePenalty = feasiblePenalty + 10.0*Ue;
        end

        switch labelCode
            case 1  % ac
                score = abs(Ie) + 0.01*max(Ue,0.0) + branchPenalty + 1e-5*Iabs;
            case 2  % vv
                score = abs(Ue) + 0.01*max(Ie,0.0) + branchPenalty - 1e-6*ctx.signT*Te;
            case 3  % av
                score = abs(Ue) + branchPenalty + 1e-6*Iabs + 0.01*max(Ie,0.0);
            case 4  % cv
                score = abs(Ie) + abs(Ue) + branchPenalty + 1e-6*ps;
            case 5  % at
                score = abs(Te - ctx.Tref) + feasiblePenalty + branchPenalty + 1e-6*Iabs;
            case 6  % tv
                score = abs(Te - ctx.Tref) + abs(Ue) + 0.05*max(Ie,0.0) + branchPenalty;
            otherwise
                score = abs(Te - ctx.Tref) + feasiblePenalty + branchPenalty;
        end

        if score < scoreBest
            scoreBest = score;
            p = x;
        end
    end
end

% ========================================================================
function [pref, boundaryCode] = solveTorqueOnFeasibleBoundary(ctx)

    Vpts = collectBoundaryPoints(ctx.xvec, ctx.yvec, ctx.Ueql, ctx);
    Cpts = collectBoundaryPoints(ctx.xvec, ctx.yvec, ctx.Ieql, ctx);

    MAX_CAND = 512;
    cand = nan(MAX_CAND,2);
    tag  = zeros(MAX_CAND,1);
    nCand = 0;

    for k = 1:size(Vpts,1)
        p = Vpts(k,:);
        if ~all(isfinite(p))
            continue;
        end
        Ie = evalGI(ctx.Ieql, p, ctx);
        T  = evalGI(ctx.Ti,   p, ctx);
        if Ie <= 1e-5 && (sign(T)==ctx.signT || abs(T)<=ctx.tolT)
            nCand = nCand + 1;
            if nCand <= MAX_CAND
                cand(nCand,:) = p;
                tag(nCand) = 1;
            end
        end
    end

    for k = 1:size(Cpts,1)
        p = Cpts(k,:);
        if ~all(isfinite(p))
            continue;
        end
        Ue = evalGI(ctx.Ueql, p, ctx);
        T  = evalGI(ctx.Ti,   p, ctx);
        if Ue <= 1e-5 && (sign(T)==ctx.signT || abs(T)<=ctx.tolT)
            nCand = nCand + 1;
            if nCand <= MAX_CAND
                cand(nCand,:) = p;
                tag(nCand) = 2;
            end
        end
    end

    pref = [NaN NaN];
    boundaryCode = int32(0);

    if nCand == 0
        return;
    end

    bestJ = inf;
    bestIdx = 0;

    for k = 1:nCand
        T = evalGI(ctx.Ti, cand(k,:), ctx);
        J = abs(T - ctx.Tref);
        if J < bestJ
            bestJ = J;
            bestIdx = k;
        end
    end

    p0 = cand(bestIdx,:);

    if tag(bestIdx) == 1
        boundaryCode = int32(1);
        pref = refineOnBoundary(p0, 1, ctx);
    else
        boundaryCode = int32(2);
        pref = refineOnBoundary(p0, 2, ctx);
    end
end

% ========================================================================
function pts = collectBoundaryPoints(xvec, yvec, G, ctx)

    MAX_PTS = 600;
    pts = nan(MAX_PTS,2);
    nPts = 0;

    nx = numel(xvec);
    ny = numel(yvec);
    tolMerge = 0.20*min([min(abs(diff(xvec))), min(abs(diff(yvec)))]);

    for r = 1:ny-1
        for c = 1:nx-1

            x1 = xvec(c);   x2 = xvec(c+1);
            y1 = yvec(r);   y2 = yvec(r+1);

            g11 = G(r,c);
            g12 = G(r,c+1);
            g21 = G(r+1,c);
            g22 = G(r+1,c+1);

            [ok, p] = edgeZeroPoint(x1,y1,g11, x2,y1,g12);
            if ok
                p = localProjectSingleCurve(p, G, xvec, yvec);
                if keepBoundaryPoint(p, pts, tolMerge, ctx)
                    nPts = nPts + 1;
                    if nPts <= MAX_PTS
                        pts(nPts,:) = p;
                    end
                end
            end

            [ok, p] = edgeZeroPoint(x2,y1,g12, x2,y2,g22);
            if ok
                p = localProjectSingleCurve(p, G, xvec, yvec);
                if keepBoundaryPoint(p, pts, tolMerge, ctx)
                    nPts = nPts + 1;
                    if nPts <= MAX_PTS
                        pts(nPts,:) = p;
                    end
                end
            end

            [ok, p] = edgeZeroPoint(x1,y2,g21, x2,y2,g22);
            if ok
                p = localProjectSingleCurve(p, G, xvec, yvec);
                if keepBoundaryPoint(p, pts, tolMerge, ctx)
                    nPts = nPts + 1;
                    if nPts <= MAX_PTS
                        pts(nPts,:) = p;
                    end
                end
            end

            [ok, p] = edgeZeroPoint(x1,y1,g11, x1,y2,g21);
            if ok
                p = localProjectSingleCurve(p, G, xvec, yvec);
                if keepBoundaryPoint(p, pts, tolMerge, ctx)
                    nPts = nPts + 1;
                    if nPts <= MAX_PTS
                        pts(nPts,:) = p;
                    end
                end
            end
        end
    end
end

% ========================================================================
function tf = keepBoundaryPoint(p, pts, tolMerge, ctx)

    tf = false;
    if ~all(isfinite(p))
        return;
    end

    T = evalGI(ctx.Ti, p, ctx);
    if ~((sign(T)==ctx.signT) || (abs(T)<=ctx.tolT))
        return;
    end

    for k = 1:size(pts,1)
        if all(isfinite(pts(k,:)))
            if hypot(pts(k,1)-p(1), pts(k,2)-p(2)) <= tolMerge
                return;
            end
        end
    end

    tf = true;
end

% ========================================================================
function [ok, p] = edgeZeroPoint(x1,y1,g1, x2,y2,g2)

    ok = false;
    p = [NaN NaN];

    if ~isfinite(g1) || ~isfinite(g2)
        return;
    end

    if g1 == 0
        ok = true;
        p = [x1 y1];
        return;
    elseif g2 == 0
        ok = true;
        p = [x2 y2];
        return;
    elseif (g1 < 0 && g2 > 0) || (g1 > 0 && g2 < 0)
        t = g1 / (g1 - g2);
        p = [x1 + t*(x2-x1), y1 + t*(y2-y1)];
        ok = true;
    end
end

% ========================================================================
function p = localProjectSingleCurve(p0, G, xvec, yvec)

    x = p0(1);
    y = p0(2);

    lbx = min(xvec); ubx = max(xvec);
    lby = min(yvec); uby = max(yvec);

    dx = min(abs(diff(xvec)));
    dy = min(abs(diff(yvec)));

    hx = max(1e-6, 0.25*dx);
    hy = max(1e-6, 0.25*dy);

    for it = 1:6
        g  = interp2_bilinear_clamped(xvec, yvec, G, x, y);
        gx = (interp2_bilinear_clamped(xvec, yvec, G, clampScalar(x+hx,lbx,ubx), y) ...
            - interp2_bilinear_clamped(xvec, yvec, G, clampScalar(x-hx,lbx,ubx), y)) / (2*hx);
        gy = (interp2_bilinear_clamped(xvec, yvec, G, x, clampScalar(y+hy,lby,uby)) ...
            - interp2_bilinear_clamped(xvec, yvec, G, x, clampScalar(y-hy,lby,uby))) / (2*hy);

        den = gx*gx + gy*gy;
        if den < 1e-16
            break;
        end

        alpha = g / den;
        x = clampScalar(x - alpha*gx, lbx, ubx);
        y = clampScalar(y - alpha*gy, lby, uby);

        if abs(g) < 1e-10
            break;
        end
    end

    p = [x y];
end

% ========================================================================
function p = refineOnBoundary(p0, btype, ctx)

    p = p0;

    for it = 1:12
        J0 = boundaryObjective(p, btype, ctx, min(ctx.xvec), max(ctx.xvec), min(ctx.yvec), max(ctx.yvec));

        dx = min(abs(diff(ctx.xvec)));
        dy = min(abs(diff(ctx.yvec)));

        cand = [ ...
            p(1)+0.5*dx, p(2);
            p(1)-0.5*dx, p(2);
            p(1), p(2)+0.5*dy;
            p(1), p(2)-0.5*dy;
            p(1)+0.25*dx, p(2)+0.25*dy;
            p(1)+0.25*dx, p(2)-0.25*dy;
            p(1)-0.25*dx, p(2)+0.25*dy;
            p(1)-0.25*dx, p(2)-0.25*dy];

        bestP = p;
        bestJ = J0;

        for k = 1:size(cand,1)
            q = cand(k,:);
            q(1) = clampScalar(q(1), min(ctx.xvec), max(ctx.xvec));
            q(2) = clampScalar(q(2), min(ctx.yvec), max(ctx.yvec));
            Jq = boundaryObjective(q, btype, ctx, min(ctx.xvec), max(ctx.xvec), min(ctx.yvec), max(ctx.yvec));
            if Jq < bestJ
                bestJ = Jq;
                bestP = q;
            end
        end

        if all(abs(bestP - p) < 1e-10)
            break;
        end
        p = bestP;
    end
end

% ========================================================================
function J = boundaryObjective(x, btype, ctx, lbx, ubx, lby, uby)

    xd = clampScalar(x(1), lbx, ubx);
    yq = clampScalar(x(2), lby, uby);
    p  = [xd yq];

    T  = evalGI(ctx.Ti,   p, ctx);
    Ie = evalGI(ctx.Ieql, p, ctx);
    Ue = evalGI(ctx.Ueql, p, ctx);

    Jt = (T - ctx.Tref)^2;

    switch btype
        case 1
            Jb = 1e6*(Ue^2) + 1e7*(max(Ie,0.0)^2);
        case 2
            Jb = 1e6*(Ie^2) + 1e7*(max(Ue,0.0)^2);
        otherwise
            Jb = 1e6*(Ie^2 + Ue^2);
    end

    Jbranch = 0.0;
    if sign(yq) ~= ctx.signT
        Jbranch = 1e5;
    end

    J = Jt + Jb + Jbranch;
end

% ========================================================================
function p = finalFeasiblePolish(p0, mode, ctx)

    p = p0;

    for it = 1:12
        J0 = finalObjective(p, mode, ctx, min(ctx.xvec), max(ctx.xvec), min(ctx.yvec), max(ctx.yvec));

        dx = min(abs(diff(ctx.xvec)));
        dy = min(abs(diff(ctx.yvec)));

        cand = [ ...
            p(1)+0.5*dx, p(2);
            p(1)-0.5*dx, p(2);
            p(1), p(2)+0.5*dy;
            p(1), p(2)-0.5*dy;
            p(1)+0.25*dx, p(2)+0.25*dy;
            p(1)+0.25*dx, p(2)-0.25*dy;
            p(1)-0.25*dx, p(2)+0.25*dy;
            p(1)-0.25*dx, p(2)-0.25*dy];

        bestP = p;
        bestJ = J0;

        for k = 1:size(cand,1)
            q = cand(k,:);
            q(1) = clampScalar(q(1), min(ctx.xvec), max(ctx.xvec));
            q(2) = clampScalar(q(2), min(ctx.yvec), max(ctx.yvec));
            Jq = finalObjective(q, mode, ctx, min(ctx.xvec), max(ctx.xvec), min(ctx.yvec), max(ctx.yvec));
            if Jq < bestJ
                bestJ = Jq;
                bestP = q;
            end
        end

        if all(abs(bestP - p) < 1e-10)
            break;
        end
        p = bestP;
    end
end

% ========================================================================
function J = finalObjective(x, mode, ctx, lbx, ubx, lby, uby)

    xd = clampScalar(x(1), lbx, ubx);
    yq = clampScalar(x(2), lby, uby);
    p  = [xd yq];

    T  = evalGI(ctx.Ti,   p, ctx);
    Ie = evalGI(ctx.Ieql, p, ctx);
    Ue = evalGI(ctx.Ueql, p, ctx);

    Jt = (T - ctx.Tref)^2;
    Jf = 1e7*(max(Ie,0.0)^2 + max(Ue,0.0)^2);

    if sign(yq) ~= ctx.signT
        Jf = Jf + 1e5;
    end

    switch mode
        case 1
            J = Jt + Jf;
        case 2
            J = Jt + 1e6*(min(Ie^2, Ue^2)) + Jf;
        case 3
            J = Jt + 1e6*(Ue^2) + 1e7*(max(Ie,0.0)^2);
        otherwise
            J = Jt + Jf;
    end
end

% ========================================================================
function z = interp2_bilinear_clamped(xvec, yvec, F, x, y)

    nx = numel(xvec);
    ny = numel(yvec);

    x = clampScalar(x, xvec(1), xvec(nx));
    y = clampScalar(y, yvec(1), yvec(ny));

    ix = findInterval(xvec, x);
    iy = findInterval(yvec, y);

    if ix >= nx
        ix = nx - 1;
    end
    if iy >= ny
        iy = ny - 1;
    end

    x1 = xvec(ix);
    x2 = xvec(ix+1);
    y1 = yvec(iy);
    y2 = yvec(iy+1);

    if x2 == x1
        tx = 0.0;
    else
        tx = (x - x1) / (x2 - x1);
    end

    if y2 == y1
        ty = 0.0;
    else
        ty = (y - y1) / (y2 - y1);
    end

    f11 = F(iy,   ix);
    f21 = F(iy,   ix+1);
    f12 = F(iy+1, ix);
    f22 = F(iy+1, ix+1);

    z1 = f11 + tx*(f21 - f11);
    z2 = f12 + tx*(f22 - f12);
    z  = z1 + ty*(z2 - z1);
end

% ========================================================================
function idx = findInterval(vec, x)

    n = numel(vec);

    if x <= vec(1)
        idx = 1;
        return;
    end

    if x >= vec(n)
        idx = n - 1;
        return;
    end

    idx = 1;
    for k = 1:n-1
        if x >= vec(k) && x <= vec(k+1)
            idx = k;
            return;
        end
    end

    idx = n - 1;
end

% ========================================================================
function y = clampScalar(x, lo, hi)
    y = min(max(x, lo), hi);
end
% ========================================================================

== matlab function Model_Linearisierung_final/Subsystem Arbeitspunktsteuerung/Drehrichtung ==
  data: T_soll input; signT output
%% Vorzeichen Drehmoment -> Festlegung Drehrichtung
function signT = fcn(T_soll)

signT = sign(T_soll);
if signT == 0
    signT = 1;
end
